simulink model "Miniproect_Control_systems"  (R2016b)
settings: Solver=VariableStepAuto  StartTime=0.0  StopTime=30.0  RelTol=1e-3
values from neighbouring files (symbols this model uses):
  B = 0.01    [WorkspaceVariables.mat]    (also in Workspace_variables.mat; matlab.m)
  b = 1    [WorkspaceVariables.mat]    (also in Workspace_variables.mat; matlab.m)
  Kephi = 1.6    [WorkspaceVariables.mat]    (also in Workspace_variables.mat; matlab.m)
  Kh = 0.5    [WorkspaceVariables.mat]    (also in Workspace_variables.mat; matlab.m)
  Kp = 0.5    [WorkspaceVariables.mat]    (also in Workspace_variables.mat; matlab.m)
  m = 0.5    [WorkspaceVariables.mat]    (also in Workspace_variables.mat; matlab.m = 1)
  Ra = 0.5    [WorkspaceVariables.mat]    (also in Workspace_variables.mat; matlab.m)
  tau_a = 0.2    [WorkspaceVariables.mat]    (also in Workspace_variables.mat; matlab.m)
  tau_m = 500    [WorkspaceVariables.mat]    (also in Workspace_variables.mat; matlab.m)
  TL = 20    [WorkspaceVariables.mat]    (also in Workspace_variables.mat; matlab.m)
undefined symbols (not defined in the file or in its folder): magnitude
libraries: simulink x1
settings Model: Creator=HP  LastModifiedBy=HP

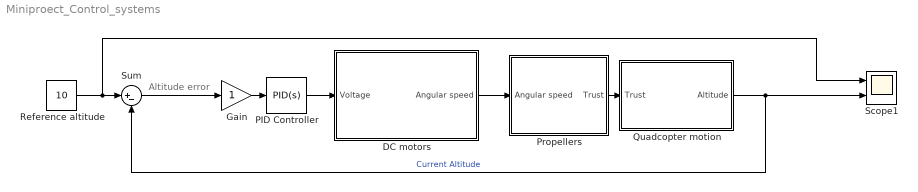
== system Miniproect_Control_systems ==
  note: Altitude error
  DC motors : Subsystem
  Gain : Gain
  PID Controller : simulink/Continuous/PID Controller  Controller=PID  TimeDomain=Continuous-time  SampleTime=-1  IntegratorMethod=Forward Euler  FilterMethod=Forward Euler  Form=Parallel  UseFilter=on  ControllerParametersSource=internal  P=0.8  I=0.5  D=0.1  N=100  InitialConditionSource=internal  InitialConditionForIntegrator=0  InitialConditionForFilter=0  ExternalReset=none  LimitOutput=off  UpperSaturationLimit=inf  LowerSaturationLimit=-inf  LinearizeAsGain=on  AntiWindupMode=none  Kb=1  TrackingMode=off  Kt=1  PParamMin=[]  PParamMax=[]  IParamMin=[]  IParamMax=[]  DParamMin=[]  DParamMax=[]  NParamMin=[]  NParamMax=[]  KbParamMin=[]  KbParamMax=[]  KtParamMin=[]  KtParamMax=[]  POutMin=[]  POutMax=[]  IOutMin=[]  IOutMax=[]  DOutMin=[]  DOutMax=[]  NOutMin=[]  NOutMax=[]  KbOutMin=[]  KbOutMax=[]  KtOutMin=[]  KtOutMax=[]  IntegratorOutMin=[]  IntegratorOutMax=[]  FilterOutMin=[]  FilterOutMax=[]  SumOutMin=[]  SumOutMax=[]  SumI1OutMin=[]  SumI1OutMax=[]  SumI2OutMin=[]  SumI2OutMax=[]  SumI3OutMin=[]  SumI3OutMax=[]  SumDOutMin=[]  SumDOutMax=[]  SaturationOutMin=[]  SaturationOutMax=[]  IntegratorContinuousStateAttributes=''  IntegratorStateMustResolveToSignalObject=off  IntegratorRTWStateStorageClass=Auto  FilterContinuousStateAttributes=''  FilterStateMustResolveToSignalObject=off  FilterRTWStateStorageClass=Auto  DifferentiatorICPrevScaledInput=0  DifferentiatorOutMin=[]  DifferentiatorOutMax=[]
  Propellers : Subsystem
  Quadcopter motion : Subsystem
  Reference altitude : Constant  Value=10
  Scope1 : Scope  NumInputPorts=2
  Sum : Sum  Inputs=|+-
  wires:
  DC motors/1(Angular speed) -> Propellers/1(Angular speed)
  Propellers/1(Trust) -> Quadcopter motion/1(Trust)
  Quadcopter motion/1(Altitude) -> Sum/2, Scope1/2  "Current Altitude"
  Sum/1 -> Gain/1
  Reference altitude/1 -> Scope1/1, Sum/1
  Gain/1 -> PID Controller/1
  PID Controller/1 -> DC motors/1(Voltage)

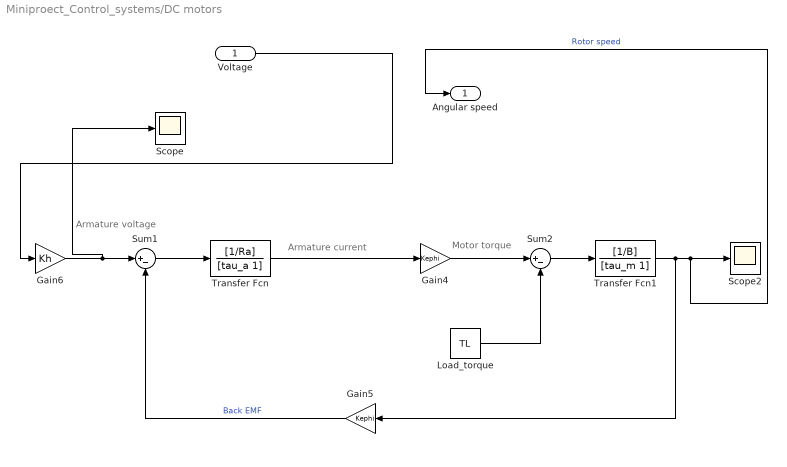
== system Miniproect_Control_systems/DC motors ==
  note: Armature voltage
  note: Motor torque
  note: Armature current
  Voltage : Inport
  Gain4 : Gain  Gain=Kephi
  Gain5 : Gain  Gain=Kephi
  Gain6 : Gain  Gain=Kh
  Load_torque : Constant  Value=TL
  Scope : Scope
  Scope2 : Scope
  Sum1 : Sum  Inputs=|+-
  Sum2 : Sum  Inputs=|+-
  Transfer Fcn : TransferFcn  Numerator=[1/Ra]  Denominator=[tau_a 1]
  Transfer Fcn1 : TransferFcn  Numerator=[1/B]  Denominator=[tau_m 1]
  Angular speed : Outport
  wires:
  Voltage/1 -> Gain6/1
  Gain5/1 -> Sum1/2  "Back EMF"
  Gain4/1 -> Sum2/1
  Load_torque/1 -> Sum2/2
  Sum2/1 -> Transfer Fcn1/1
  Sum1/1 -> Transfer Fcn/1
  Transfer Fcn1/1 -> Gain5/1, Angular speed/1, Scope2/1  "Rotor speed"
  Transfer Fcn/1 -> Gain4/1
  Gain6/1 -> Scope/1, Sum1/1

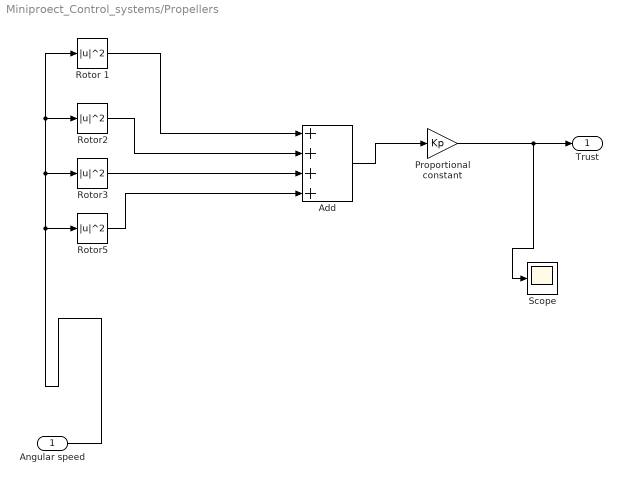
== system Miniproect_Control_systems/Propellers ==
  Angular speed : Inport
  Add : Sum  Inputs=++++
  Proportional constant : Gain  Gain=Kp
  Rotor 1 : Math  Operator=magnitude^2  SaturateOnIntegerOverflow=on
  Rotor2 : Math  Operator=magnitude^2  SaturateOnIntegerOverflow=on
  Rotor3 : Math  Operator=magnitude^2  SaturateOnIntegerOverflow=on
  Rotor5 : Math  Operator=magnitude^2  SaturateOnIntegerOverflow=on
  Scope : Scope
  Trust : Outport
  wires:
  Rotor5/1 -> Add/4
  Proportional constant/1 -> Scope/1, Trust/1
  Rotor2/1 -> Add/2
  Add/1 -> Proportional constant/1
  Angular speed/1 -> Rotor5/1, Rotor3/1, Rotor2/1, Rotor 1/1
  Rotor 1/1 -> Add/1
  Rotor3/1 -> Add/3

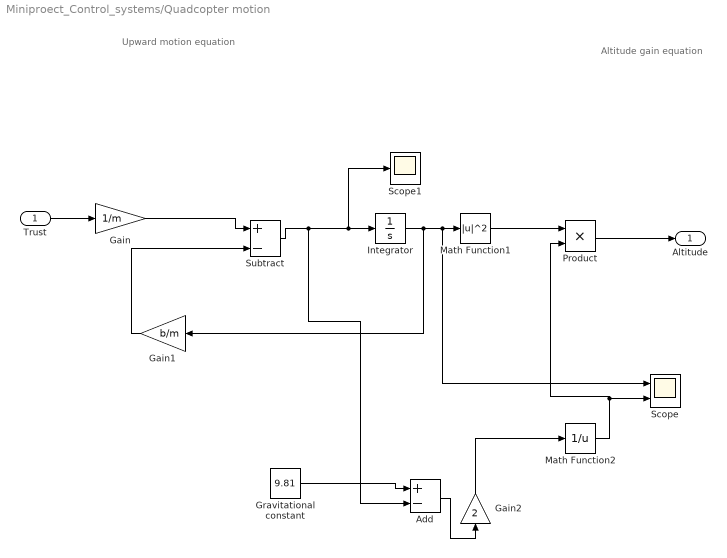
== system Miniproect_Control_systems/Quadcopter motion ==
  note: Altitude gain equation
  note: Upward motion equation
  Trust : Inport
  Add : Sum  Inputs=+-
  Gain : Gain  Gain=1/m
  Gain1 : Gain  Gain=b/m
  Gain2 : Gain  Gain=2
  Gravitational constant : Constant  Value=9.81
  Integrator : Integrator
  Math Function1 : Math  Operator=magnitude^2  SaturateOnIntegerOverflow=on
  Math Function2 : Math  Operator=reciprocal  SaturateOnIntegerOverflow=on
  Product : Product
  Scope : Scope  NumInputPorts=2
  Scope1 : Scope
  Subtract : Sum  Inputs=+-
  Altitude : Outport
  wires:
  Math Function1/1 -> Product/1
  Gain1/1 -> Subtract/2
  Integrator/1 -> Scope/1, Math Function1/1, Gain1/1
  Subtract/1 -> Add/2, Scope1/1, Integrator/1
  Trust/1 -> Gain/1
  Product/1 -> Altitude/1
  Gain/1 -> Subtract/1
  Add/1 -> Gain2/1
  Gravitational constant/1 -> Add/1
  Math Function2/1 -> Product/2, Scope/2
  Gain2/1 -> Math Function2/1
